simulink model "test_fft"  (R2017b)
settings: Solver=FixedStepDiscrete  StartTime=0.0  StopTime=10  FixedStep=0.001  RelTol=1e-3  EnableMultiTasking=on
libraries: Library_SignalGeneration x2, simulink x1
settings Model: Creator=Keith  LastModifiedBy=Keith
settings OptimizationCC: LifeSpan=inf
settings DebuggingCC: SFUnexpectedBacktrackingDiag=warning  SFNoUnconditionalDefaultTransitionDiag=warning  SFExecutionAtInitializationDiag=none
settings CodeAppCC: StateflowObjectComments=on
settings GRTTargetCC: TargetLangStandard=C89/C90 (ANSI)  GeneratePreprocessorConditionals=Disable all
settings ConfigComp: CovMetricSettings=dw  CovHtmlReporting=on  CovSaveCumulativeToWorkspaceVar=on  CovSaveSingleToWorkspaceVar=on  CovExternalEMLEnable=off

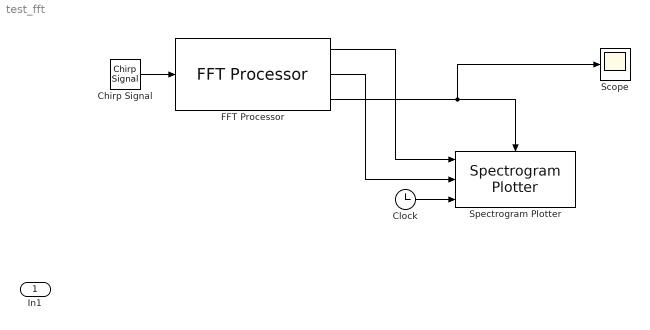
== system test_fft ==
  In1 : Inport
  Chirp Signal : simulink/Sources/Chirp Signal  f1=0.1  T=10  f2=500
  Clock : Clock
  FFT Processor : Library_SignalGeneration/FFT Processor  BUFFSIZE=256  FFTSIZE=256  OVLP_PRCNT=0
  Scope : Scope
  Spectrogram Plotter : Library_SignalGeneration/Spectrogram Plotter  nRows=64  complexFFT=off  Fs=1000  Zo=50  cMin=-60  cMax=10
      settings: AttributesFormatString=|
      | Fs=%<Fs> | Zo=%<Zo>
      | Displays %<nRows> Rows
  wires:
  FFT Processor/1 -> Spectrogram Plotter/1
  FFT Processor/2 -> Spectrogram Plotter/2
  FFT Processor/3 -> Spectrogram Plotter/Trigger, Scope/1
  Chirp Signal/1 -> FFT Processor/1
  Clock/1 -> Spectrogram Plotter/3
